simulink model "MPC_AVC"  (Simulink 8.5)
settings: Solver=ode5  StartTime=0.0  StopTime=Total_t_sim  FixedStep=dt  RelTol=1e-3
values from neighbouring files (symbols this model uses):
  A = F    [DMPC_AVC.m]    (also in identified.mat = [-0.773996386153 -96.4009703983 0 0 0 0 96.979553948 -1.6354)
  A_cons = [L_m;-L_m]    [DMPC_AVC.m]
  B = G    [DMPC_AVC.m]    (also in identified.mat = [-0.230745598618  -0.153904745996; 0.0612777559553  0.060617)
  Bg = Bg(:,1:2)    [DMPC_AVC.m]
  C = H    [DMPC_AVC.m]    (also in identified.mat = [-23.1554338545 9.56281796835 0.435674513054 -0.46619419818 )
  coefs = coefs(1,2:end)    [DMPC_AVC.m]
  dt = 0.001    [DMPC_AVC.m]
  Hg = Bg(:,3)    [DMPC_AVC.m]
  L1 = dlqr(A',C',1e-5*eye(size(A)),1e-7)'    [DMPC_AVC.m]
  Lf = Kalman_Gain(A,C,Qf,Rf,Pf,Nsim,nout)    [DMPC_AVC.m]
  Ps = 1e1    (= 10)    [DMPC_AVC.m]
  Rs = 1e-1    (= 0.1)    [DMPC_AVC.m]
  Total_t_sim = Total_t-10*dt    (= 4.99)    [DMPC_AVC.m]
  u_bound = [u_max;-u_min]    [DMPC_AVC.m]
undefined symbols (not defined in the file or in its folder): Ag, Cg, L_m, omega, psi
libraries: simulink x1
settings Model: Creator=Farhang  LastModifiedBy=p4wp4w
settings DebuggingCC: SolverPrmCheckMsg=warning  FcnCallInpInsideContextMsg=UseLocalSettings

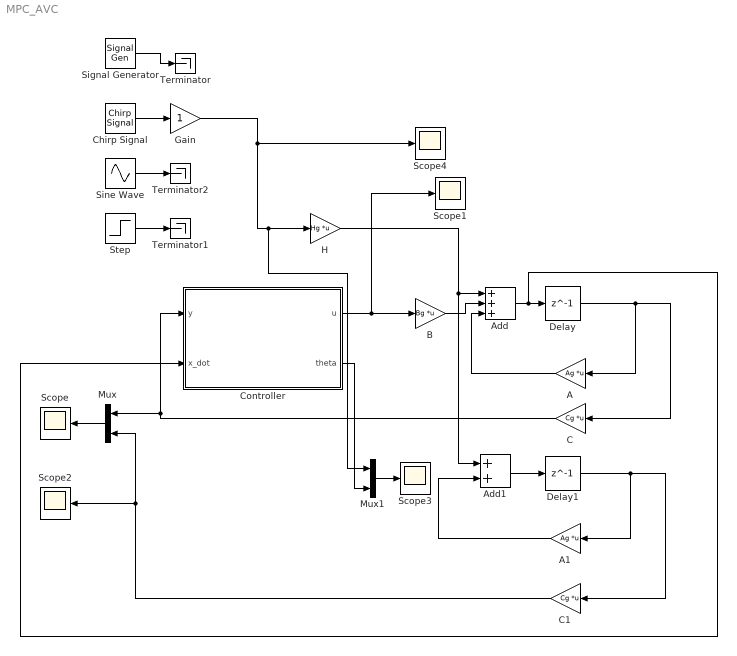
== system MPC_AVC ==
  A : Gain  Gain=Ag  Multiplication=Matrix(K*u)
  A1 : Gain  Gain=Ag  Multiplication=Matrix(K*u)
  Add : Sum  Inputs=+++
  Add1 : Sum
  B : Gain  Gain=Bg  Multiplication=Matrix(K*u)
  C : Gain  Gain=Cg  Multiplication=Matrix(K*u)
  C1 : Gain  Gain=Cg  Multiplication=Matrix(K*u)
  Chirp Signal : simulink/Sources/Chirp Signal  f1=5  T=Total_t_sim  f2=90
  Controller : Subsystem
  Delay : Delay  DelayLength=1  InitialCondition=0
  Delay1 : Delay  DelayLength=1  InitialCondition=0
  Gain : Gain
  H : Gain  Gain=Hg  Multiplication=Matrix(K*u)
  Mux : Mux  Inputs=2
  Mux1 : Mux  Inputs=2
  Scope{,1..4} (5 alike) : Scope
      Scope settings: ShowLegends=on  YMin=-0.7  YMax=0.6
      Scope1 settings: ShowLegends=on  YMin=-0.0007  YMax=0.0007  SaveName=ScopeData2
      Scope2 settings: ShowLegends=on  YMin=-0.005  YMax=0.0045  SaveName=ScopeData3
      Scope3 settings: ShowLegends=on  YMin=-1  YMax=1  SaveName=ScopeData4
      Scope4 settings: ShowLegends=on  YMin=-0.0007  YMax=0.0007  SaveName=ScopeData5
  Signal Generator : SignalGenerator  WaveForm=square
  Sine Wave : Sin  Frequency=96.7  SampleTime=dt
  Step : Step  Time=2*dt  SampleTime=0
  Terminator : Terminator
  Terminator1 : Terminator
  Terminator2 : Terminator
  wires:
  Delay/1 -> A/1, C/1
  Add/1 -> Controller/2(x_dot), Delay/1
  C/1 -> Mux/1, Controller/1(y)
  A/1 -> Add/3
  H/1 -> Add1/1, Add/1
  Delay1/1 -> C1/1, A1/1
  Add1/1 -> Delay1/1
  A1/1 -> Add1/2
  Mux/1 -> Scope/1
  C1/1 -> Scope2/1, Mux/2
  Step/1 -> Terminator1/1
  Mux1/1 -> Scope3/1
  Controller/2(theta) -> Mux1/2
  B/1 -> Add/2
  Controller/1(u) -> Scope1/1, B/1
  Sine Wave/1 -> Terminator2/1
  Chirp Signal/1 -> Gain/1
  Gain/1 -> Scope4/1, Mux1/1, H/1
  Signal Generator/1 -> Terminator/1

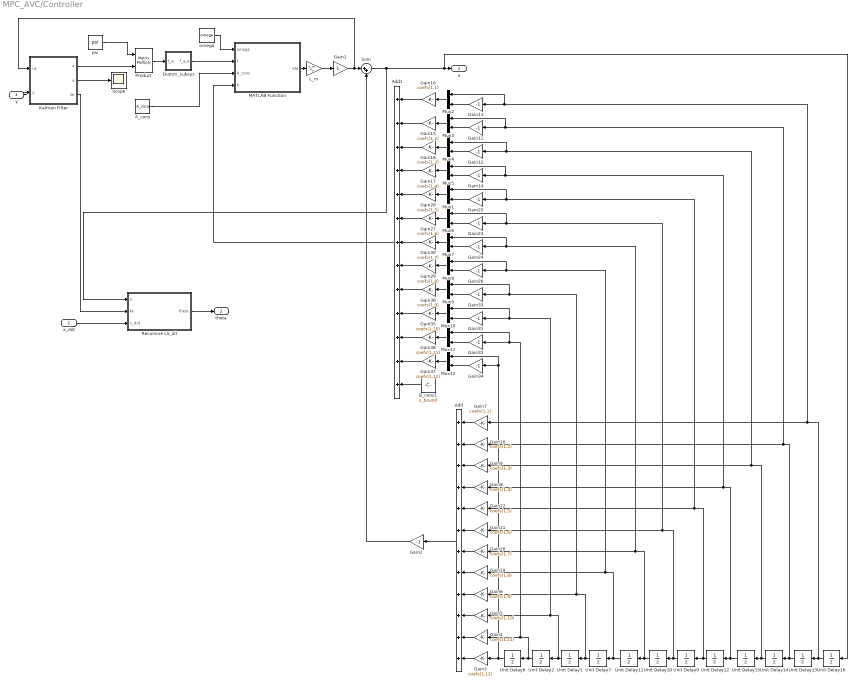
== system MPC_AVC/Controller ==
  y : Inport
  x_dot : Inport  Port=2
  A_cons : Constant  Value=A_cons  SampleTime=dt
  Add : Sum  Inputs=++++++++++++
  Add1 : Sum  Inputs=+++++++++++++
  B_cons1 : Constant  Value=u_bound
  Dumm_subsys : Subsystem
  Gain1 : Gain
  Gain10 : Gain  Gain=coefs(1,2)
  Gain{2,11..14,23..26,31..34} (13 alike) : Gain  Gain=-1
  Gain15 : Gain  Gain=coefs(1,2)
  Gain16 : Gain  Gain=coefs(1,1)
  Gain17 : Gain  Gain=coefs(1,4)
  Gain18 : Gain  Gain=coefs(1,3)
  Gain19 : Gain  Gain=coefs(1,8)
  Gain20 : Gain  Gain=coefs(1,7)
  Gain21 : Gain  Gain=coefs(1,6)
  Gain22 : Gain  Gain=coefs(1,5)
  Gain27 : Gain  Gain=coefs(1,6)
  Gain28 : Gain  Gain=coefs(1,5)
  Gain29 : Gain  Gain=coefs(1,8)
  Gain3 : Gain  Gain=coefs(1,12)
  Gain30 : Gain  Gain=coefs(1,7)
  Gain35 : Gain  Gain=coefs(1,10)
  Gain36 : Gain  Gain=coefs(1,9)
  Gain37 : Gain  Gain=coefs(1,12)
  Gain38 : Gain  Gain=coefs(1,11)
  Gain4 : Gain  Gain=coefs(1,11)
  Gain5 : Gain  Gain=coefs(1,10)
  Gain6 : Gain  Gain=coefs(1,9)
  Gain7 : Gain  Gain=coefs(1,1)
  Gain8 : Gain  Gain=coefs(1,4)
  Gain9 : Gain  Gain=coefs(1,3)
  Kalman Filter : Subsystem  TreatAsAtomicUnit=on
  L_m : Gain  Gain=L_m  Multiplication=Matrix(K*u)
  MATLAB Function : MATLAB Function  TreatAsAtomicUnit=on
  Mux{1..12} (12 alike) : Mux  Inputs=2
  Product : Product  Multiplication=Matrix(*)  RndMeth=Zero
  Recursive LS_all : Subsystem
  Scope : Scope
      settings: YMin=-0.000155  YMax=-6.5e-05
  Sum : Sum  Inputs=|++
  Unit Delay{1..2,6..7,9..16} (12 alike) : UnitDelay  SampleTime=dt
  omega : Constant  Value=omega  SampleTime=dt
  psi : Constant  Value=psi  SampleTime=dt
  u : Outport
  theta : Outport  Port=2
  wires:
  MATLAB Function/1(eta) -> L_m/1
  L_m/1 -> Gain1/1
  omega/1 -> MATLAB Function/1(omega)
  A_cons/1 -> MATLAB Function/3(A_cons)
  psi/1 -> Product/1
  y/1 -> Kalman Filter/2(y)
  Gain7/1 -> Add/1
  Gain9/1 -> Add/3
  Gain8/1 -> Add/4
  Gain13/1 -> Mux2/2
  Gain11/1 -> Mux3/2
  Gain12/1 -> Mux4/2
  Gain14/1 -> Mux5/2
  Mux2/1 -> Gain16/1
  Mux3/1 -> Gain15/1
  Mux4/1 -> Gain18/1
  Mux5/1 -> Gain17/1
  Gain16/1 -> Add1/1
  Gain15/1 -> Add1/2
  Gain18/1 -> Add1/3
  Gain17/1 -> Add1/4
  Add/1 -> Gain2/1
  Gain10/1 -> Add/2
  Product/1 -> Dumm_subsys/1(f_in)
  Dumm_subsys/1(f_out) -> MATLAB Function/2(f)
  Kalman Filter/1(X) -> Product/2
  Kalman Filter/2(e) -> Scope/1
  Gain1/1 -> Sum/1, Kalman Filter/1(us)
  Unit Delay2/1 -> Mux11/1, Gain32/1, Gain4/1, Unit Delay6/1
  Unit Delay1/1 -> Mux10/1, Gain31/1, Gain5/1, Unit Delay2/1
  Unit Delay7/1 -> Gain6/1, Mux9/1, Gain33/1, Unit Delay1/1
  Unit Delay11/1 -> Mux8/1, Gain26/1, Gain19/1, Unit Delay7/1
  Unit Delay10/1 -> Mux7/1, Gain24/1, Gain20/1, Unit Delay11/1
  Unit Delay9/1 -> Mux6/1, Gain23/1, Gain21/1, Unit Delay10/1
  Unit Delay12/1 -> Mux1/1, Gain25/1, Gain22/1, Unit Delay9/1
  Unit Delay15/1 -> Gain14/1, Mux5/1, Gain8/1, Unit Delay12/1
  Unit Delay14/1 -> Mux4/1, Gain12/1, Gain9/1, Unit Delay15/1
  Unit Delay13/1 -> Mux3/1, Gain11/1, Gain10/1, Unit Delay14/1
  Unit Delay16/1 -> Mux2/1, Gain13/1, Gain7/1, Unit Delay13/1
  Gain3/1 -> Add/12
  Unit Delay6/1 -> Gain34/1, Mux12/1, Gain3/1
  Gain4/1 -> Add/11
  Gain5/1 -> Add/10
  Gain6/1 -> Add/9
  Gain19/1 -> Add/8
  Gain20/1 -> Add/7
  Gain21/1 -> Add/6
  Gain22/1 -> Add/5
  B_cons1/1 -> Add1/13
  Gain25/1 -> Mux1/2
  Gain23/1 -> Mux6/2
  Gain24/1 -> Mux7/2
  Gain26/1 -> Mux8/2
  Mux1/1 -> Gain28/1
  Mux6/1 -> Gain27/1
  Mux7/1 -> Gain30/1
  Mux8/1 -> Gain29/1
  Gain33/1 -> Mux9/2
  Gain31/1 -> Mux10/2
  Gain32/1 -> Mux11/2
  Gain34/1 -> Mux12/2
  Mux9/1 -> Gain36/1
  Mux10/1 -> Gain35/1
  Mux11/1 -> Gain38/1
  Mux12/1 -> Gain37/1
  Gain28/1 -> Add1/5
  Gain27/1 -> Add1/6
  Gain30/1 -> Add1/7
  Gain29/1 -> Add1/8
  Gain36/1 -> Add1/9
  Gain35/1 -> Add1/10
  Gain38/1 -> Add1/11
  Gain37/1 -> Add1/12
  Sum/1 -> Recursive LS_all/1(u), Unit Delay16/1, u/1
  Kalman Filter/3(kk) -> Recursive LS_all/2(kk)
  Add1/1 -> MATLAB Function/4(b)
  Gain2/1 -> Sum/2
  Recursive LS_all/1(theta) -> theta/1
  x_dot/1 -> Recursive LS_all/3(x_dot)

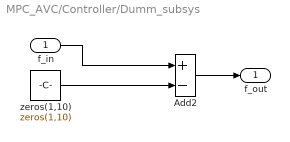
== system MPC_AVC/Controller/Dumm_subsys ==
  f_in : Inport
  Add2 : Sum  Inputs=+-
  zeros(1,10) : Constant  Value=zeros(1,10)  SampleTime=dt
  f_out : Outport
  wires:
  f_in/1 -> Add2/1
  Add2/1 -> f_out/1
  zeros(1,10)/1 -> Add2/2

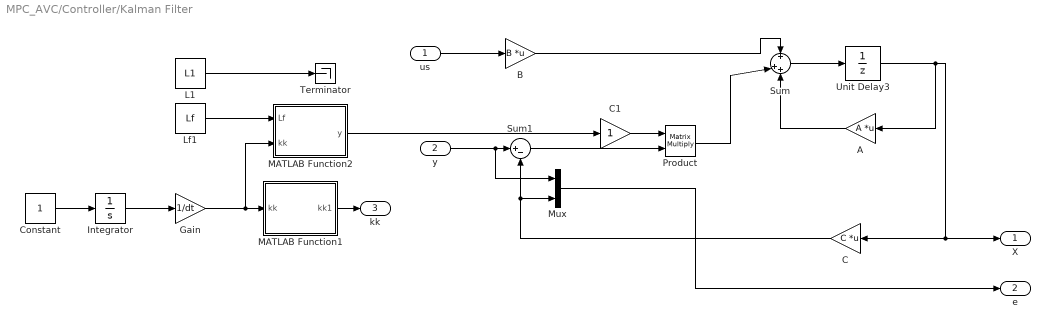
== system MPC_AVC/Controller/Kalman Filter ==
  us : Inport
  y : Inport  Port=2
  A : Gain  Gain=A  Multiplication=Matrix(K*u)
  B : Gain  Gain=B  Multiplication=Matrix(K*u)
  C : Gain  Gain=C  Multiplication=Matrix(K*u)
  C1 : Gain
  Constant : Constant
  Gain : Gain  Gain=1/dt
  Integrator : Integrator
  L1 : Constant  Value=L1
  Lf1 : Constant  Value=Lf
  MATLAB Function1 : MATLAB Function  TreatAsAtomicUnit=on
  MATLAB Function2 : MATLAB Function  TreatAsAtomicUnit=on
  Mux : Mux  Inputs=2
  Product : Product  Multiplication=Matrix(*)  RndMeth=Zero
  Sum : Sum  Inputs=+|++
  Sum1 : Sum  Inputs=|+-
  Terminator : Terminator
  Unit Delay3 : UnitDelay  SampleTime=dt
  X : Outport
  e : Outport  Port=2
  kk : Outport  Port=3
  wires:
  Unit Delay3/1 -> A/1, X/1, C/1
  A/1 -> Sum/3
  Sum/1 -> Unit Delay3/1
  us/1 -> B/1
  B/1 -> Sum/1
  C/1 -> Mux/2, Sum1/2
  y/1 -> Mux/1, Sum1/1
  Sum1/1 -> Product/2
  Product/1 -> Sum/2
  Constant/1 -> Integrator/1
  Integrator/1 -> Gain/1
  Lf1/1 -> MATLAB Function2/1(Lf)
  Gain/1 -> MATLAB Function1/1(kk), MATLAB Function2/2(kk)
  L1/1 -> Terminator/1
  MATLAB Function2/1(y) -> C1/1
  C1/1 -> Product/1
  Mux/1 -> e/1
  MATLAB Function1/1(kk1) -> kk/1

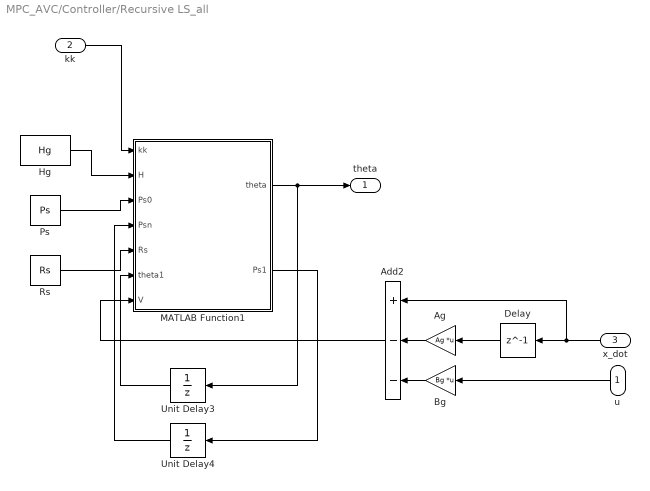
== system MPC_AVC/Controller/Recursive LS_all ==
  u : Inport
  kk : Inport  Port=2
  x_dot : Inport  Port=3
  Add2 : Sum  Inputs=+--
  Ag : Gain  Gain=Ag  Multiplication=Matrix(K*u)
  Bg : Gain  Gain=Bg  Multiplication=Matrix(K*u)
  Delay : Delay  DelayLength=1  InitialCondition=0
  Hg : Constant  Value=Hg  SampleTime=dt
  MATLAB Function1 : MATLAB Function  TreatAsAtomicUnit=on
  Ps : Constant  Value=Ps  SampleTime=dt
  Rs : Constant  Value=Rs  SampleTime=dt
  Unit Delay3 : UnitDelay  SampleTime=dt
  Unit Delay4 : UnitDelay  SampleTime=dt
  theta : Outport
  wires:
  MATLAB Function1/2(Ps1) -> Unit Delay4/1
  MATLAB Function1/1(theta) -> theta/1, Unit Delay3/1
  kk/1 -> MATLAB Function1/1(kk)
  Ps/1 -> MATLAB Function1/3(Ps0)
  Unit Delay3/1 -> MATLAB Function1/6(theta1)
  Hg/1 -> MATLAB Function1/2(H)
  Rs/1 -> MATLAB Function1/5(Rs)
  Unit Delay4/1 -> MATLAB Function1/4(Psn)
  x_dot/1 -> Add2/1, Delay/1
  Delay/1 -> Ag/1
  Ag/1 -> Add2/2
  Bg/1 -> Add2/3
  u/1 -> Bg/1
  Add2/1 -> MATLAB Function1/7(V)

== matlab function Controller/MATLAB Function ==
  data: omega input double; eta output double; f input double; A_cons input double; b input double
function eta=QPomegaild(omega,f,A_cons,b)

[n1,m1]=size(A_cons);
% eta=-omega\f;
eta=-inv(omega)*f;
kk=0;
for i=1:n1
    if (A_cons(i,:)*eta>b(i)) 
        kk=kk+1;
    else
        kk=kk+0;
    end
end
if (kk==0)
    return
end
P=A_cons*(omega\A_cons');
d=(A_cons*(omega\f)+b);
[n,m]=size(d);
x_ini=zeros(n,m);
lambda=x_ini;
% al=10;
for km=1:38

%find tomegae elements in tomegae solution vector one by one
% km could be larger if tomegae Lagranger multiplier omegaas a slow
% convergence rate.
    lambda_p=lambda;
    for i=1:n
        w= P(i,:)*lambda-P(i,i)*lambda(i,1);
        w=w+d(i,1);
        la=-w/P(i,i);
        lambda(i,1)=max(0,la);
    end
    
    al=(lambda-lambda_p)'*(lambda-lambda_p);
    if (al<10e-8)
        break;
    end
 end
eta=-omega\f -omega\A_cons'*lambda;

== matlab function Controller/Kalman Filter/MATLAB Function2 ==
  data: y output double; Lf input double; kk input double
function y = fcn(Lf,kk)
%#codegen

kk = floor(kk)+1;

y = Lf(:,kk);

== matlab function Controller/Kalman Filter/MATLAB Function1 ==
  data: kk1 output double; kk input double
function kk1 = fcn(kk)
%#codegen

kk1 = floor(kk)+1;

== matlab function Controller/Recursive LS_all/MATLAB Function1 ==
  data: kk input double; H input double; Ps0 input double; Psn input double; Rs input double; theta1 input double; theta output double; Ps1 output double; V input double
function [theta,Ps1] = fcn(kk,H,Ps0,Psn,Rs,theta1,V)
%#codegen
if (kk==1)
    Ps = Ps0;
    Ks=(Ps*H')/(H*Ps*H'+Rs);
    theta=theta1+Ks*(V-H*theta1);
    Ps1=(eye(1)-Ks*H)*Ps*(eye(1)-Ks*H)'+Ks*Rs*Ks';
else
    Ps = Psn;
    Ks=(Ps*H')/(H*Ps*H'+Rs);
    theta=theta1+Ks*(V-H*theta1);
    Ps1=(eye(1)-Ks*H)*Ps*(eye(1)-Ks*H)'+Ks*Rs*Ks';
end
